simulink model "test"  (R2015a)
settings: Solver=ode45  StartTime=0.0  StopTime=10.0  RelTol=1e-3
values from neighbouring files (symbols this model uses):
  b = 0.2    [Data.mat]
  j = 0.01    [Data.mat]
  K = 0.1    [Data.mat]
  L = 0.5    [Data.mat]
  R = 1    [Data.mat]
undefined symbols (not defined in the file or in its folder): fdesignblkfcn, gcbh
settings Model: Creator=adelgayed60  LastModifiedBy=adelgayed60

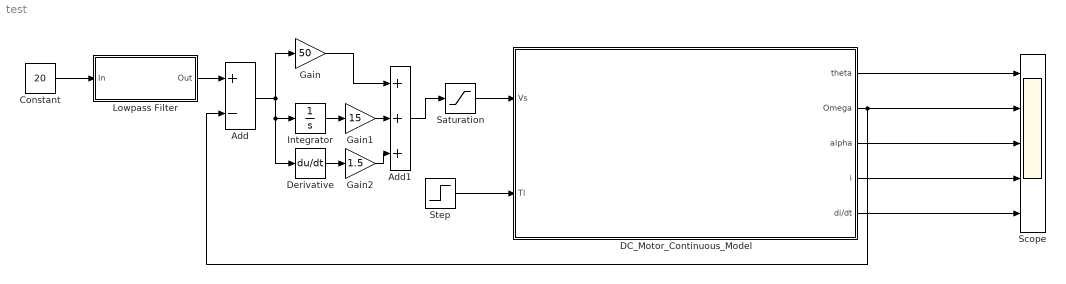
== system test ==
  Add : Sum  Inputs=+-
  Add1 : Sum  Inputs=+++
  Constant : Constant  Value=20
  DC_Motor_Continuous_Model : Subsystem
  Derivative : Derivative
  Gain : Gain  Gain=50
  Gain1 : Gain  Gain=15
  Gain2 : Gain  Gain=1.5
  Integrator : Integrator
  Lowpass Filter : Subsystem  DialogController=fdesignblkfcn  InitFcn=fdesignblkfcn(gcbh, {'InitFcn'});  mask(Lowpass Filter){}
      mask help: Design a lowpass filter
      settings: CopyFcn=fdesignblkfcn(gcbh, {'CopyFcn'});
      mask Help: helpview(mapfilelocation('dsp'), 'dsplowpassfilter');
      mask Display: disp('Lowpass')
  Saturation : Saturate  UpperLimit=100  LowerLimit=0
  Scope : Scope  NumInputPorts=5
      settings: YMin=-5~-5~-5~-5~-5  YMax=5~5~5~5~5
  Step : Step  Time=5  SampleTime=0
  wires:
  Add/1 -> Derivative/1, Integrator/1, Gain/1
  Constant/1 -> Lowpass Filter/1(In)
  Saturation/1 -> DC_Motor_Continuous_Model/1(Vs)
  Step/1 -> DC_Motor_Continuous_Model/2(Tl)
  DC_Motor_Continuous_Model/4(i) -> Scope/4
  DC_Motor_Continuous_Model/1(theta) -> Scope/1
  DC_Motor_Continuous_Model/2(Omega) -> Add/2, Scope/2
  DC_Motor_Continuous_Model/3(alpha) -> Scope/3
  DC_Motor_Continuous_Model/5(di/dt) -> Scope/5
  Gain/1 -> Add1/1
  Add1/1 -> Saturation/1
  Integrator/1 -> Gain1/1
  Gain1/1 -> Add1/2
  Derivative/1 -> Gain2/1
  Gain2/1 -> Add1/3
  Lowpass Filter/1(Out) -> Add/1

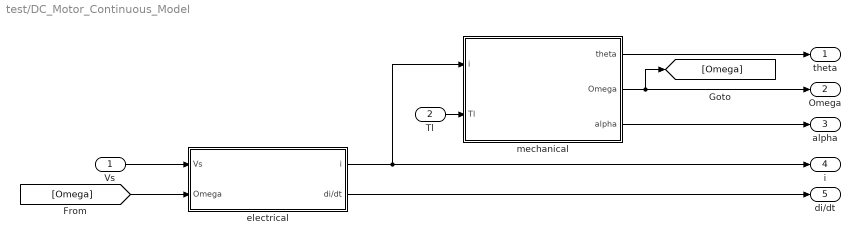
== system test/DC_Motor_Continuous_Model ==
  Vs : Inport
  Tl : Inport  Port=2
  electrical : Subsystem
  mechanical : Subsystem
  theta : Outport
  Omega : Outport  Port=2
  alpha : Outport  Port=3
  i : Outport  Port=4
  di/dt : Outport  Port=5
  wires:
  Vs/1 -> electrical/1(Vs)
  mechanical/1(theta) -> theta/1
  [Omega] -> electrical/2(Omega)
  mechanical/2(Omega) -> Omega/1, [Omega]
  Tl/1 -> mechanical/2(Tl)
  electrical/1(i) -> i/1, mechanical/1(i)
  electrical/2(di/dt) -> di/dt/1
  mechanical/3(alpha) -> alpha/1

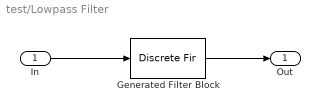
== system test/Lowpass Filter ==
  In : Inport
  Generated Filter Block : DiscreteFir  Tag=BlockMethodSubSystem  Coefficients=[-0.001565521559079915 0.0051422462219556271 -0.012763948200316441 0.02688191136851514 -0.051583684792804056 0.095933131376735231 -0.19191236389001448 0.62959541978942535 0.62959541978942535 -0.19191236389001448 0.095933131376735231 -0.051583684792804056 0.02688191136851514 -0.012763948200316441 0.0051422462219556271 -0.001565521559079915]  InputProcessing=Columns as channels (frame based)
  Out : Outport
  wires:
  In/1 -> Generated Filter Block/1
  Generated Filter Block/1 -> Out/1

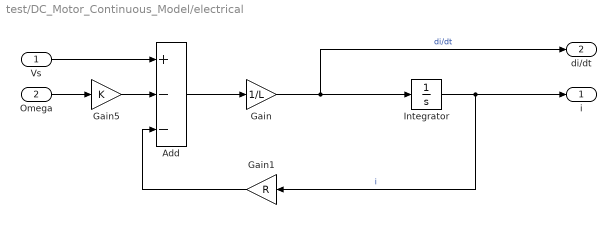
== system test/DC_Motor_Continuous_Model/electrical ==
  Vs : Inport
  Omega : Inport  Port=2
  Add : Sum  Inputs=+--
  Gain : Gain  Gain=1/L
  Gain1 : Gain  Gain=R
  Gain5 : Gain  Gain=K
  Integrator : Integrator
  i : Outport
  di/dt : Outport  Port=2
  wires:
  Gain/1 -> di/dt/1, Integrator/1  "di/dt"
  Gain1/1 -> Add/3
  Integrator/1 -> i/1, Gain1/1  "i"
  Add/1 -> Gain/1
  Vs/1 -> Add/1
  Omega/1 -> Gain5/1
  Gain5/1 -> Add/2

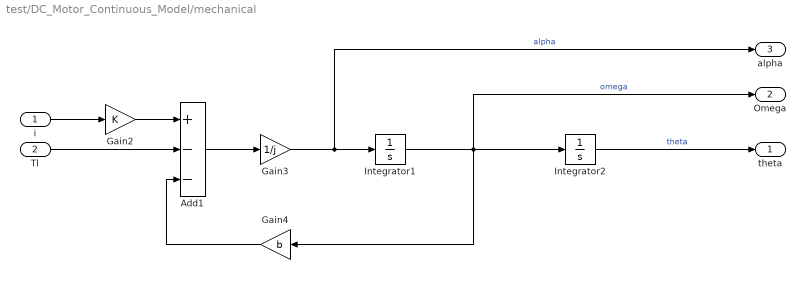
== system test/DC_Motor_Continuous_Model/mechanical ==
  i : Inport
  Tl : Inport  Port=2
  Add1 : Sum  Inputs=+--
  Gain2 : Gain  Gain=K
  Gain3 : Gain  Gain=1/j
  Gain4 : Gain  Gain=b
  Integrator1 : Integrator
  Integrator2 : Integrator
  theta : Outport
  Omega : Outport  Port=2
  alpha : Outport  Port=3
  wires:
  i/1 -> Gain2/1
  Gain3/1 -> alpha/1, Integrator1/1  "alpha"
  Integrator1/1 -> Omega/1, Gain4/1, Integrator2/1  "omega"
  Integrator2/1 -> theta/1  "theta"
  Gain4/1 -> Add1/3
  Add1/1 -> Gain3/1
  Gain2/1 -> Add1/1
  Tl/1 -> Add1/2
